simulink model "sampleModel1411"  (R2023a)
settings: Solver=VariableStepAuto  StartTime=0.0  StopTime=10.0  RelTol=1e-3
libraries: hdlsllib x4, simulink x1
settings Model: Creator=user1  LastModifiedBy=user1

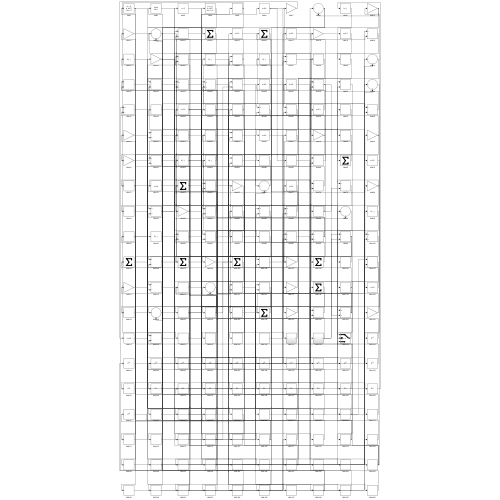
[thumbnail: Simulink's stored preview of the top-level diagram]
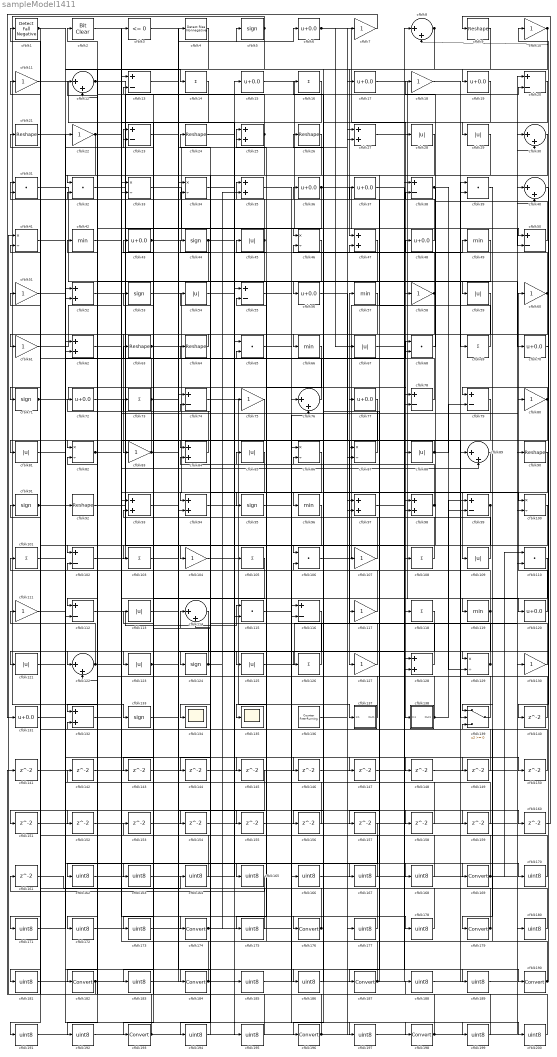
== system sampleModel1411 ==
  cfblk1 : hdlsllib/Logic and Bit Operations/Detect Fall Negative  vinit=0  OutDataTypeStr=boolean
  cfblk{7,10..11,18,22,51,58,60..61,75,80,83,104,107,111,117,127,130} (18 alike) : Gain
  cfblk{33..34,41,46,82,86..87,100,129} (9 alike) : Product  Inputs=*/  RndMeth=Zero  SaturateOnIntegerOverflow=on
  cfblk{14,16,69,73,101,103,105,108,118,126} (10 alike) : Sum  Inputs=+
  cfblk{13,20,23,38,50,55,74,78..79,99,102,112,116} (13 alike) : Sum  Inputs=+-
  cfblk{31..32,39,65,68,106,110,115} (8 alike) : DotProduct  OutDataTypeStr=Inherit: Inherit via internal rule
  cfblk{28..29,45,54,59,67,81,85,88,109,113,121,123,125} (14 alike) : Abs  SaturateOnIntegerOverflow=off
  cfblk{8,12,30,40,76,89,114,122} (8 alike) : Sum  Inputs=|++
  cfblk{42,49,57,66,96,119} (6 alike) : MinMax
  cfblk{6,15,17,19,36..37,43,48,56,70,72,77,120,131} (14 alike) : Bias  Bias=0.0  SaturateOnIntegerOverflow=off
  cfblk{5,44,53,71,91,95,124,133} (8 alike) : Signum
  cfblk{25,27,35,47,52,62,84,93..94,97..98,128,132} (13 alike) : Sum
  cfblk134 : Scope
  cfblk135 : Scope
  cfblk136 : hdlsllib/Sources/Counter Free-Running  NumBits=16  tsamp=-1
  cfblk137 : Subsystem
      settings: LibrarySourceBlock=|
      | hdlsllib/Ports &
      | Subsystems/Subsystem
  cfblk138 : Subsystem
      settings: LibrarySourceBlock=|
      | hdlsllib/Ports &
      | Subsystems/Subsystem
  cfblk139 : Switch  SaturateOnIntegerOverflow=off  InputSameDT=off
  cfblk{140..161} (22 alike) : Delay  SampleTime=1
  cfblk{162..168,170..173,175,177..178,180..181,183,185..186,188..189,191..192,194..195,197,199..200} (28 alike) : DataTypeConversion  OutDataTypeStr=uint8  SaturateOnIntegerOverflow=off  RndMeth=Floor
  cfblk{169,174,176,179,182,184,187,190,193,196,198} (11 alike) : DataTypeConversion  SaturateOnIntegerOverflow=off  RndMeth=Floor
  cfblk2 : simulink/Logic and Bit Operations/Bit Clear  iBit=0
      settings: LibrarySourceBlock=|
      | hdlsllib/Logic and Bit
      | Operations/Bit Clear
  cfblk{9,21,24,26,63..64,90,92} (8 alike) : Reshape
  cfblk3 : hdlsllib/Logic and Bit Operations/Compare To Zero  relop=<=  OutDataTypeStr=boolean
  cfblk4 : hdlsllib/Logic and Bit Operations/Detect Rise Nonnegative  vinit=0  OutDataTypeStr=boolean
  wires:
  cfblk97/1 -> cfblk190/1
  cfblk38/1 -> cfblk102/1, cfblk129/2
  cfblk8/1 -> cfblk47/1, cfblk122/2
  cfblk17/1 -> cfblk59/1
  cfblk113/1 -> cfblk6/1
  cfblk20/1 -> cfblk29/1
  cfblk74/1 -> cfblk137/1(In1)
  cfblk102/1 -> cfblk20/2
  cfblk12/1 -> cfblk104/1, cfblk132/1
  cfblk15/1 -> cfblk50/1
  cfblk127/1 -> cfblk57/1
  cfblk44/1 -> cfblk158/1, cfblk192/1, cfblk197/1
  cfblk60/1 -> cfblk83/1, cfblk37/1
  cfblk40/1 -> cfblk129/1
  cfblk120/1 -> cfblk60/1
  cfblk107/1 -> cfblk43/1
  cfblk5/1 -> cfblk133/1, cfblk112/2
  cfblk61/1 -> cfblk3/1
  cfblk82/1 -> cfblk94/1, cfblk80/1
  cfblk52/1 -> cfblk27/1
  cfblk27/1 -> cfblk119/1
  cfblk53/1 -> cfblk100/1
  cfblk31/1 -> cfblk70/1
  cfblk36/1 -> cfblk138/1(In1), cfblk152/1
  cfblk112/1 -> cfblk115/1
  cfblk108/1 -> cfblk36/1
  cfblk111/1 -> cfblk169/1
  cfblk64/1 -> cfblk61/1
  cfblk6/1 -> cfblk58/1, cfblk67/1
  cfblk131/1 -> cfblk22/1
  cfblk11/1 -> cfblk75/1
  cfblk26/1 -> cfblk134/1
  cfblk126/1 -> cfblk31/1
  cfblk2/1 -> cfblk84/1
  cfblk58/1 -> cfblk26/1, cfblk94/2
  cfblk49/1 -> cfblk56/1
  cfblk106/1 -> cfblk28/1
  cfblk136/1 -> cfblk17/1
  cfblk98/1 -> cfblk24/1, cfblk74/2
  cfblk80/1 -> cfblk79/1, cfblk163/1
  cfblk138/1(Out1) -> cfblk54/1, cfblk99/1, cfblk99/2
  cfblk39/1 -> cfblk179/1
  cfblk45/1 -> cfblk12/2, cfblk173/1
  cfblk88/1 -> cfblk82/1, cfblk79/2
  cfblk92/1 -> cfblk106/1
  cfblk9/1 -> cfblk66/1
  cfblk75/1 -> cfblk124/1
  cfblk119/1 -> cfblk125/1, cfblk44/1
  cfblk56/1 -> cfblk88/1
  cfblk124/1 -> cfblk63/1, cfblk93/2, cfblk35/2
  cfblk18/1 -> cfblk69/1
  cfblk99/1 -> cfblk112/1, cfblk151/1
  cfblk22/1 -> cfblk32/1, cfblk78/2, cfblk145/1
  cfblk91/1 -> cfblk68/1, cfblk189/1
  cfblk33/1 -> cfblk46/1
  cfblk132/1 -> cfblk49/1
  cfblk117/1 -> cfblk21/1
  cfblk50/1 -> cfblk18/1
  cfblk83/1 -> cfblk5/1, cfblk81/1
  cfblk73/1 -> cfblk11/1, cfblk122/1, cfblk155/1
  cfblk123/1 -> cfblk126/1, cfblk186/1
  cfblk63/1 -> cfblk127/1, cfblk25/2
  cfblk42/1 -> cfblk174/1
  cfblk84/1 -> cfblk32/2
  cfblk76/1 -> cfblk12/1
  cfblk7/1 -> cfblk131/1
  cfblk13/1 -> cfblk176/1
  cfblk69/1 -> cfblk47/2
  cfblk125/1 -> cfblk40/1
  cfblk101/1 -> cfblk23/1
  cfblk128/1 -> cfblk87/1
  cfblk71/1 -> cfblk78/1, cfblk121/1
  cfblk14/1 -> cfblk103/1
  cfblk110/1 -> cfblk139/1
  cfblk32/1 -> cfblk50/2
  cfblk139/1 -> cfblk31/2
  cfblk109/1 -> cfblk35/1
  cfblk90/1 -> cfblk196/1
  cfblk29/1 -> cfblk52/2
  cfblk94/1 -> cfblk107/1
  cfblk59/1 -> cfblk62/2
  cfblk47/1 -> cfblk135/1
  cfblk137/1(Out1) -> cfblk64/1
  cfblk35/1 -> cfblk76/1
  cfblk25/1 -> cfblk2/1, cfblk115/2
  cfblk66/1 -> cfblk95/1
  cfblk48/1 -> cfblk23/2
  cfblk79/1 -> cfblk98/2
  cfblk72/1 -> cfblk139/2
  cfblk129/1 -> cfblk123/1, cfblk84/2, cfblk73/1
  cfblk104/1 -> cfblk48/1
  cfblk122/1 -> cfblk101/1, cfblk89/2
  cfblk103/1 -> cfblk128/2
  cfblk34/1 -> cfblk65/1
  cfblk89/1 -> cfblk109/1
  cfblk86/1 -> cfblk184/1
  cfblk16/1 -> cfblk33/2
  cfblk114/1 -> cfblk193/1
  cfblk130/1 -> cfblk85/1
  cfblk43/1 -> cfblk7/1, cfblk120/1, cfblk146/1
  cfblk68/1 -> cfblk38/2
  cfblk10/1 -> cfblk8/2, cfblk19/1
  cfblk1/1 -> cfblk14/1, cfblk71/1
  cfblk3/1 -> cfblk108/1
  cfblk41/1 -> cfblk198/1
  cfblk78/1 -> cfblk25/1
  cfblk23/1 -> cfblk96/1
  cfblk62/1 -> cfblk117/1
  cfblk118/1 -> cfblk182/1
  cfblk30/1 -> cfblk187/1
  cfblk87/1 -> cfblk16/1
  cfblk70/1 -> cfblk140/1
  cfblk140/1 -> cfblk102/2
  cfblk141/1 -> cfblk68/2
  cfblk142/1 -> cfblk87/2
  cfblk105/1 -> cfblk143/1
  cfblk143/1 -> cfblk38/1
  cfblk100/1 -> cfblk144/1
  cfblk146/1 -> cfblk27/2
  cfblk133/1 -> cfblk147/1
  cfblk147/1 -> cfblk89/1
  cfblk81/1 -> cfblk148/1
  cfblk148/1 -> cfblk20/1
  cfblk37/1 -> cfblk149/1
  cfblk149/1 -> cfblk1/1
  cfblk24/1 -> cfblk150/1
  cfblk150/1 -> cfblk98/1
  cfblk151/1 -> cfblk76/2
  cfblk152/1 -> cfblk74/1
  cfblk153/1 -> cfblk40/2
  cfblk85/1 -> cfblk154/1
  cfblk155/1 -> cfblk128/1
  cfblk19/1 -> cfblk156/1
  cfblk156/1 -> cfblk33/1
  cfblk28/1 -> cfblk157/1
  cfblk158/1 -> cfblk52/1
  cfblk67/1 -> cfblk159/1
  cfblk159/1 -> cfblk46/2
  cfblk95/1 -> cfblk160/1
  cfblk160/1 -> cfblk9/1
  cfblk4/1 -> cfblk162/1
  cfblk162/1 -> cfblk15/1
  cfblk163/1 -> cfblk4/1
  cfblk161/1 -> cfblk164/1
  cfblk164/1 -> cfblk62/1
  cfblk21/1 -> cfblk165/1
  cfblk165/1 -> cfblk161/1
  cfblk55/1 -> cfblk166/1
  cfblk166/1 -> cfblk110/2
  cfblk51/1 -> cfblk167/1
  cfblk167/1 -> cfblk55/1
  cfblk65/1 -> cfblk168/1
  cfblk168/1 -> cfblk55/2
  cfblk169/1 -> cfblk132/2, cfblk110/1
  cfblk121/1 -> cfblk170/1
  cfblk170/1 -> cfblk111/1
  cfblk116/1 -> cfblk171/1
  cfblk171/1 -> cfblk92/1
  cfblk157/1 -> cfblk172/1
  cfblk172/1 -> cfblk116/1
  cfblk173/1 -> cfblk116/2
  cfblk174/1 -> cfblk34/2, cfblk105/1
  cfblk77/1 -> cfblk175/1
  cfblk175/1 -> cfblk42/1
  cfblk176/1 -> cfblk65/2, cfblk51/1
  cfblk177/1 -> cfblk13/1
  cfblk93/1 -> cfblk178/1
  cfblk178/1 -> cfblk13/2
  cfblk179/1 -> cfblk106/2, cfblk91/1
  cfblk180/1 -> cfblk39/1
  cfblk145/1 -> cfblk181/1
  cfblk181/1 -> cfblk39/2
  cfblk182/1 -> cfblk141/1, cfblk34/1
  cfblk96/1 -> cfblk183/1
  cfblk183/1 -> cfblk118/1
  cfblk184/1 -> cfblk153/1, cfblk130/1, cfblk8/1
  cfblk144/1 -> cfblk185/1
  cfblk185/1 -> cfblk86/1
  cfblk186/1 -> cfblk86/2
  cfblk187/1 -> cfblk100/2, cfblk77/1, cfblk93/1
  cfblk188/1 -> cfblk30/1
  cfblk189/1 -> cfblk30/2
  cfblk190/1 -> cfblk45/1, cfblk139/3, cfblk53/1, cfblk10/1
  cfblk57/1 -> cfblk191/1
  cfblk191/1 -> cfblk97/1
  cfblk192/1 -> cfblk97/2
  cfblk193/1 -> cfblk180/1, cfblk82/2, cfblk72/1
  cfblk46/1 -> cfblk194/1
  cfblk194/1 -> cfblk114/1
  cfblk154/1 -> cfblk195/1
  cfblk195/1 -> cfblk114/2
  cfblk196/1 -> cfblk177/1, cfblk113/1
  cfblk197/1 -> cfblk90/1
  cfblk198/1 -> cfblk188/1, cfblk142/1
  cfblk54/1 -> cfblk199/1
  cfblk199/1 -> cfblk41/1
  cfblk115/1 -> cfblk200/1
  cfblk200/1 -> cfblk41/2

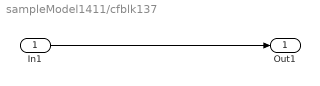
== system sampleModel1411/cfblk137 ==
  In1 : Inport
  Out1 : Outport
  wires:
  In1/1 -> Out1/1

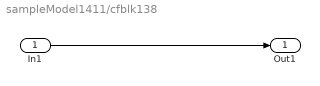
== system sampleModel1411/cfblk138 ==
  In1 : Inport
  Out1 : Outport
  wires:
  In1/1 -> Out1/1
